simulink model "test_SOC_SOH"  (R2024a)
settings: Solver=VariableStepAuto  StartTime=0.0  StopTime=3600*24*7  RelTol=1e-3
values from neighbouring files (symbols this model uses):
  cell_capacity_nominal = 116.0    [CellDictionary.sldd]    (also in Gotion116CellDictionary.sldd)
  cycling_N_cycles : value not decoded    [TestDictionary.sldd]
  cycling_Q_change : value not decoded    [TestDictionary.sldd]
  lower_SOC = 0.0    [TestDictionary.sldd]
  R0_charge = 0.0011762548470330098 0.00082374580425955042 0.000528220046847626 0.00036375900896813311 0.0010441063780583621 0.00072163805067231468 0.00050986311152455624 0.00035574030260694049 0.0010321299216333078 0.00071105826266249655 0.00048266835826310457 0.00035372216488075841 0.001024720077996646 0.00069001121087368356 0.00048481817133183287 0.00034648647498852108 0.001011799939308299 0.0006697964359567    [CellDictionary.sldd]    (also in Gotion116CellDictionary.sldd)
  R0_discharge = 0.0011713156680267826 0.00080379131757867114 0.00053584971835591568 0.00037332457313021659 0.0011487629449379545 0.00077055056377129218 0.00052328698011887883 0.00035835507369999319 0.0011266444560462821 0.0007386844798434178 0.00050172364877783509 0.0003498356430994423 0.0010850138368129973 0.00069989297656780321 0.00047637432800705728 0.00034196489943770015 0.0010386918064711587 0.00065988337212    [CellDictionary.sldd]    (also in Gotion116CellDictionary.sldd)
  R1_charge = 0.00046991497657839924 0.0010779816764740048 0.00013720748025427109 0.00054498496863974164 0.00046376138253324481 0.00066376489201272156 0.00013720748025427109 0.00018528267520728436 0.00041621818829090906 0.00049349026745049 0.00020770204245624234 0.00018502550552971592 0.00041621893904479396 0.00049355079737852447 0.00036345316071937457 0.00018502550475278616 0.00030655167459223354 0.00020155261    [CellDictionary.sldd]    (also in Gotion116CellDictionary.sldd)
  R1_discharge = 0.00062343910396692745 0.00088344565476029683 0.000473998175802181 0.00030361323697364274 0.00034635505775940415 0.00063103261054306924 0.0003646139813862931 0.00025301103081136895 0.00024739646982814583 0.00052586050878589109 0.00030384498448857757 0.00023001002801033537 0.00022490588166195074 0.00047805500798717366 0.00027622271317143414 0.00021905716953365273 0.00022546269140634405 0.0003001510    [CellDictionary.sldd]    (also in Gotion116CellDictionary.sldd)
  R2_charge = 0.0013071970907491625 0.0011565350014947392 0.00094770363400168442 0.00027803074491849166 0.0011296066387324344 0.00079964133367552734 0.000585621349864987 0.00040094855176715479 0.00096825717163721565 0.00071275071905804873 0.00050086266287882315 0.00022186351951754667 0.000858047601085684 0.00068372107937354906 0.00048716119953890212 0.00021951334854306714 0.00082371775210131749 0.00056587719522    [CellDictionary.sldd]    (also in Gotion116CellDictionary.sldd)
  R2_discharge = 0.0082023616629522487 0.00477357645651923 0.0013535754139770782 0.00071689319983068869 0.0027341205543174162 0.0015911921521730766 0.00084598463373567378 0.00044805824989418042 0.0013670602771587081 0.00088399564009615365 0.00060427473838262416 0.00037338187491181703 0.00091137351810580548 0.00073666303341346137 0.00050356228198552015 0.0003556017856303019 0.00092980892733805819 0.0007515620058816    [CellDictionary.sldd]    (also in Gotion116CellDictionary.sldd)
  R3_charge = 0.0022791079484232404 0.00076358338365525792 0.0012549156736722906 0.00058631541275341111 0.0012276125164720909 0.00076358338365525792 0.00035824943217463234 0.00076079543468179163 0.0011171764499634 0.00069457337864931717 0.00035533139001579984 0.00094337886181821427 0.0006671085355807189 0.00046891528577433023 0.00033689307388307945 0.00072524071500878735 0.00058184070468519759 0.000371910545995    [CellDictionary.sldd]    (also in Gotion116CellDictionary.sldd)
  R3_discharge = 0.5961801788597515 0.049373498218042031 0.0017231068556688191 0.0031135501588106253 0.05961801788597515 0.0098746996436084068 0.00086155342783440954 0.0017297500882281251 0.0059618017885975146 0.0019749399287216814 0.00057436895188960632 0.0012355357773058038 0.000993633631432919 0.00065831330957389386 0.0004418222706843125 0.0011232143430052761 0.0013277019879200426 0.00096507261335108377 0.00043    [CellDictionary.sldd]    (also in Gotion116CellDictionary.sldd)
  soc_init = 0.31    [SOC_tester.m]    (also in TestDictionary.sldd = 0.5
                real
                1.0 1.0
           )
  Ts = 1.0    [EstimatorsDictionary.sldd]    (also in batteryStateTransition.m = u(3))
  upper_SOC = 1.0    [TestDictionary.sldd]
undefined symbols (not defined in the file or in its folder): R, thermal_mass
libraries: fl_lib x8, nesl_utility x4, simulink x3, BatteryEstimators x2, batteryecm_lib x1, batt_lib x1
settings Model: DataDictionary=TestDictionary.sldd  Creator=mmackenzie  LastModifiedBy=mmackenzie

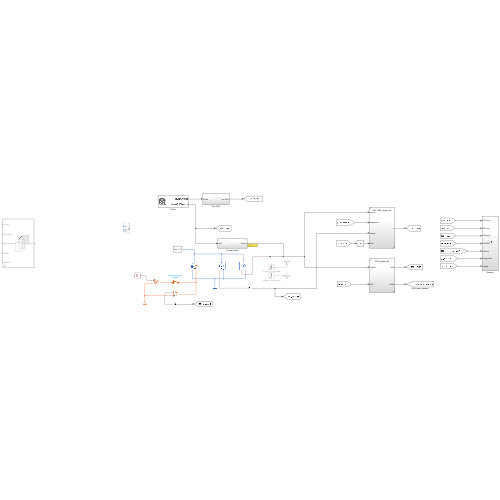
[thumbnail: Simulink's stored preview of the top-level diagram]
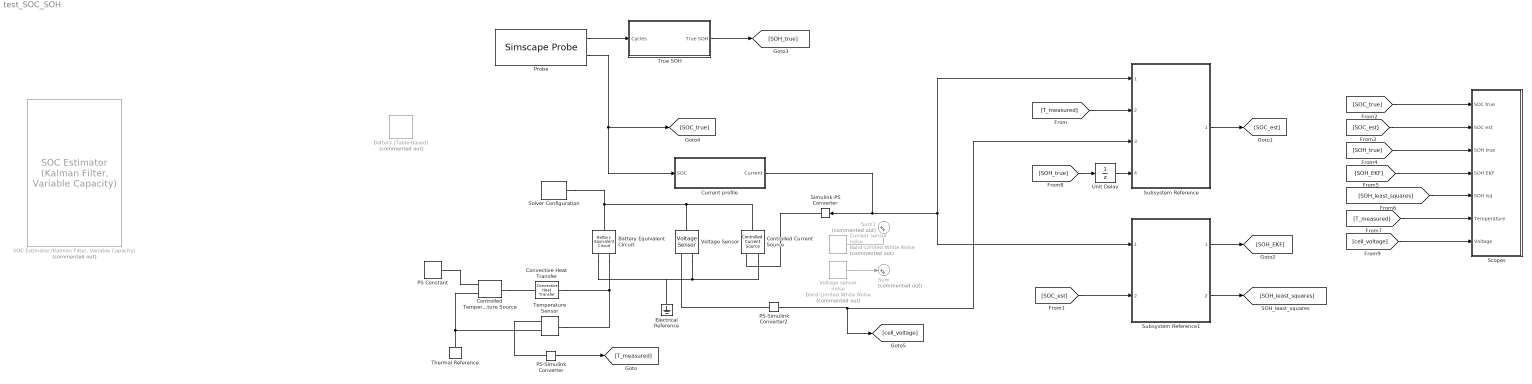
== system test_SOC_SOH ==
  Battery (Table-Based) : batteryecm_lib/Battery (Table-Based)  Commented=on  SOC_vec=SOC_vec  T_dependence=simscape.enum.tablebattery.temperature_dependence.yes  prm_dir=simscape.enum.tablebattery.prm_dir.noCurrentDirectionality  T_vec=T_vec K  V0_mat=V0_mat V  V0_vec=[3.5057, 3.566, 3.6337, 3.7127, 3.9259, 4.0777, 4.1928] V  V_range=[0, inf] V  R0_mat=R0_mat Ohm  R0_vec=[.0085, .0085, .0087, .0082, .0083, .0085, .0085] Ohm  R0_dis_mat=[.0117, .0085, .009; .011, .0085, .009; .0114, .0087, .0092; .0107, .0082, .0088; .0107, .0083, .0091; .0113, .0085, .0089; .0116, .0085, .0089] Ohm  R0_dis_vec=[.0085, .0085, .0087, .0082, .0083, .0085, .0085] Ohm  R0_ch_mat=[.0117, .0085, .009; .011, .0085, .009; .0114, .0087, .0092; .0107, .0082, .0088; .0107, .0083, .0091; .0113, .0085, .0089; .0116, .0085, .0089] Ohm  R0_ch_vec=[.0085, .0085, .0087, .0082, .0083, .0085, .0085] Ohm  AH=cell_capacity_init A*hr  prm_leak=simscape.enum.tablebattery.prm_leak.disabled  Rleak_vec=[8000, 7000, 6000] Ohm  Rleak=7e3 Ohm  extrapolation_option=simscape.enum.extrapolation.linear  SOC_port=simscape.enum.tablebattery.enable.yes  prm_dyn=simscape.enum.tablebattery.prm_dyn.rc1  R1_mat=R1_mat Ohm  R1_vec=[.0029, .0024, .0026, .0016, .0023, .0018, .0017] Ohm  tau1_mat=tau1_mat s  tau1_vec=[36, 45, 105, 29, 77, 33, 39] s  R2_mat=[.0109, .0029, .0013; .0069, .0024, .0012; .0047, .0026, .0013; .0034, .0016, .001; .0033, .0023, .0014; .0033, .0018, .0011; .0028, .0017, .0011] Ohm  R2_vec=[.0029, .0024, .0026, .0016, .0023, .0018, .0017] Ohm  tau2_mat=[20, 36, 39; 31, 45, 39; 109, 105, 61; 36, 29, 26; 59, 77, 67; 40, 33, 29; 25, 39, 33] s  tau2_vec=[36, 45, 105, 29, 77, 33, 39] s  R3_mat=[.0109, .0029, .0013; .0069, .0024, .0012; .0047, .0026, .0013; .0034, .0016, .001; .0033, .0023, .0014; .0033, .0018, .0011; .0028, .0017, .0011] Ohm  R3_vec=[.0029, .0024, .0026, .0016, .0023, .0018, .0017] Ohm  tau3_mat=[20, 36, 39; 31, 45, 39; 109, 105, 61; 36, 29, 26; 59, 77, 67; 40, 33, 29; 25, 39, 33] s  tau3_vec=[36, 45, 105, 29, 77, 33, 39] s  R4_mat=[.0109, .0029, .0013; .0069, .0024, .0012; .0047, .0026, .0013; .0034, .0016, .001; .0033, .0023, .0014; .0033, .0018, .0011; .0028, .0017, .0011] Ohm  R4_vec=[.0029, .0024, .0026, .0016, .0023, .0018, .0017] Ohm  tau4_mat=[20, 36, 39; 31, 45, 39; 109, 105, 61; 36, 29, 26; 59, 77, 67; 40, 33, 29; 25, 39, 33] s  tau4_vec=[36, 45, 105, 29, 77, 33, 39] s  R5_mat=[.0109, .0029, .0013; .0069, .0024, .0012; .0047, .0026, .0013; .0034, .0016, .001; .0033, .0023, .0014; .0033, .0018, .0011; .0028, .0017, .0011] Ohm  R5_vec=[.0029, .0024, .0026, .0016, .0023, .0018, .0017] Ohm  tau5_mat=[20, 36, 39; 31, 45, 39; 109, 105, 61; 36, 29, 26; 59, 77, 67; 40, 33, 29; 25, 39, 33] s  tau5_vec=[36, 45, 105, 29, 77, 33, 39] s  prm_fade=simscape.enum.tablebattery.prm_fade.tableN  N0=100  dV0=0  dR0=0  dAH=0  dRleak=0  dR1=0  dR2=0  dR3=0  dR4=0  dR5=0  N0vec=N0vec  Tfadevec=[298.15, 323.15] K  dV0vec=[0, 0, 0, 0, 0]  dR0vec=[0, 0, 0, 0, 0]  dAHvec=dAHvec  dRleakvec=[0, 0, 0, 0]  dR1vec=[0, 0, 0, 0, 0]  dR2vec=[0, 0, 0, 0]  dR3vec=[0, 0, 0, 0]  dR4vec=[0, 0, 0, 0]  dR5vec=[0, 0, 0, 0]  dV0mat=[0, 0; 0, 0; 0, 0; 0, 0]  dR0mat=[0, 0; 0, 0; 0, 0; 0, 0]  dAHmat=[0, 0; 0, 0; 0, 0; 0, 0]  dRleakmat=[0, 0; 0, 0; 0, 0; 0, 0]  dR1mat=[0, 0; 0, 0; 0, 0; 0, 0]  dR2mat=[0, 0; 0, 0; 0, 0; 0, 0]  dR3mat=[0, 0; 0, 0; 0, 0; 0, 0]  dR4mat=[0, 0; 0, 0; 0, 0; 0, 0]  dR5mat=[0, 0; 0, 0; 0, 0; 0, 0]  prm_age_modeling=simscape.enum.tablebattery.prm_age_modeling.equation  storage_dt_age_vec=[0] d  storage_T_age_vec=[273] K  prm_age_OCV=simscape.enum.tablebattery.prm_age_OCV.OCV  OCV_age=0.9  SOC_age=0.6  prm_age_resistance=simscape.enum.tablebattery.prm_age.disabled  OCV_scaling_age_resistance=2.2134e6  OCV_offset_age_resistance=1.632e6  temp_exp_age_resistance=0.515833569 V  t_exp_age_resistance=0.75  T_age_vec_resistance=[273.15, 298.15, 323.15] K  dt_age_vec_resistance=[0, 90, 180, 270] d  dR0_age_vec=[0, 0, 0]  t_meas_dR0_age=100 d  dR0_age_mat=[0, 0, 0; 0, 0, 0; 0, 0, 0; 0, 0, 0]  prm_age_capacity=simscape.enum.tablebattery.prm_age.disabled  OCV_scaling_age_capacity=1.5097e07  OCV_offset_age_capacity=8.3625e06  temp_exp_age_capacity=0.6011 V  t_exp_age_capacity=0.75  T_age_vec_capacity=[273.15, 298.15, 323.15] K  dt_age_vec_capacity=[0, 90, 180, 270] d  dAH_age_vec=[0, 0, 0]  t_meas_dAH_age=100 d  dAH_age_mat=[0, 0, 0; 0, 0, 0; 0, 0, 0; 0, 0, 0]  thermal_port=simscape.enum.thermaleffects.model  temperature=298.15 K  thermal_mass=thermal_mass*1.5 J/K  i_specify=off  i_priority=None  i=0 A  i_nominal_specify=off  i_nominal_value=1  i_nominal_unit=A  v_specify=off  v_priority=None  v=0 V  v_nominal_specify=off  v_nominal_value=1  v_nominal_unit=V  stateOfCharge_specify=on  stateOfCharge_priority=High  stateOfCharge=initialSOC  stateOfCharge_nominal_specify=off  stateOfCharge_nominal_value=1  stateOfCharge_nominal_unit=1  num_cycles_specify=off  num_cycles_priority=High  num_cycles=0  num_cycles_nominal_specify=off  num_cycles_nominal_value=1  num_cycles_nominal_unit=1  cell_temperature_specify=off  cell_temperature_priority=High  cell_temperature=298.15 K  cell_temperature_nominal_specify=off  cell_temperature_nominal_value=1  cell_temperature_nominal_unit=K
      settings: LibrarySourceBlock=|
      | batt_lib/Cells/Battery
      | (Table-Based)
  Battery Equivalent Circuit : batt_lib/Cells/Battery Equivalent Circuit  BatteryCapacity=cell_capacity_nominal A*hr  ThermalModel=simscape.battery.enum.cells.BatteryThermalModel.LumpedThermalMass  ExtrapolationMethod=simscape.enum.extrapolation.nearest  EnableFaultExotherm=false  TriggerTemperature=350 K  SOCBreakpoints=OCV_SOC  TemperatureBreakpoints=OCV_T degC  OpenCircuitVoltage=[3.5057, 3.566, 3.6337, 3.7127, 3.9259, 4.0777, 4.1928] V  OpenCircuitVoltageThermal=OCV_V V  VoltageRange=[2.8, 4.25] V  HysteresisModel=simscape.battery.enum.cells.HysteresisModel.none  MaximumHysteresisVoltage=[0, 0, 0, 0, 0, 0, 0] V  InstantaneousHysteresisVoltage=[0, 0, 0, 0, 0, 0, 0] V  HysteresisRate=0.1  MaximumHysteresisVoltageThermal=[0, 0, 0; 0, 0, 0; 0, 0, 0; 0, 0, 0; 0, 0, 0; 0, 0, 0; 0, 0, 0] V  InstantaneousHysteresisVoltageThermal=[0, 0, 0; 0, 0, 0; 0, 0, 0; 0, 0, 0; 0, 0, 0; 0, 0, 0; 0, 0, 0] V  HysteresisRateThermal=0.1  ResistanceSOCBreakpoints=ECM_SOC'  ResistanceTemperatureBreakpoints=ECM_T' degC  CurrentDirectionality=simscape.battery.enum.cells.BatteryEnable.Enabled  R0=[.0085, .0085, .0087, .0082, .0083, .0085, .0085] Ohm  R0Thermal=[.0117, .0085, .009; .011, .0085, .009; .0114, .0087, .0092; .0107, .0082, .0088; .0107, .0083, .0091; .0113, .0085, .0089; .0116, .0085, .0089] Ohm  DischargeR0=[.0085, .0085, .0087, .0082, .0083, .0085, .0085] Ohm  ChargeR0=[.0085, .0085, .0087, .0082, .0083, .0085, .0085] Ohm  ChargeR0Thermal=R0_charge' Ohm  DischargeR0Thermal=R0_discharge' Ohm  SelfDischargeResistor=simscape.battery.enum.cells.BatteryEnable.Disabled  SelfDischargeR=7e3 Ohm  SelfDischargeRThermal=[8000, 7000, 6000] Ohm  RCPairs=simscape.battery.enum.cells.RCPairs.rc3  R1=[.0029, .0024, .0026, .0016, .0023, .0018, .0017] Ohm  Tau1=[36, 45, 105, 29, 77, 33, 39] s  R2=[.0029, .0024, .0026, .0016, .0023, .0018, .0017] Ohm  Tau2=[36, 45, 105, 29, 77, 33, 39] s  R3=[.0029, .0024, .0026, .0016, .0023, .0018, .0017] Ohm  Tau3=[36, 45, 105, 29, 77, 33, 39] s  DischargeR1=[.0029, .0024, .0026, .0016, .0023, .0018, .0017] Ohm  DischargeTau1=[36, 45, 105, 29, 77, 33, 39] s  ChargeR1=[.0029, .0024, .0026, .0016, .0023, .0018, .0017] Ohm  ChargeTau1=[36, 45, 105, 29, 77, 33, 39] s  DischargeR2=[.0029, .0024, .0026, .0016, .0023, .0018, .0017] Ohm  DischargeTau2=[36, 45, 105, 29, 77, 33, 39] s  ChargeR2=[.0029, .0024, .0026, .0016, .0023, .0018, .0017] Ohm  ChargeTau2=[36, 45, 105, 29, 77, 33, 39] s  DischargeR3=[.0029, .0024, .0026, .0016, .0023, .0018, .0017] Ohm  DischargeTau3=[36, 45, 105, 29, 77, 33, 39] s  ChargeR3=[.0029, .0024, .0026, .0016, .0023, .0018, .0017] Ohm  ChargeTau3=[36, 45, 105, 29, 77, 33, 39] s  R1Thermal=[.0109, .0029, .0013; .0069, .0024, .0012; .0047, .0026, .0013; .0034, .0016, .001; .0033, .0023, .0014; .0033, .0018, .0011; .0028, .0017, .0011] Ohm  Tau1Thermal=[20, 36, 39; 31, 45, 39; 109, 105, 61; 36, 29, 26; 59, 77, 67; 40, 33, 29; 25, 39, 33] s  R2Thermal=[.0109, .0029, .0013; .0069, .0024, .0012; .0047, .0026, .0013; .0034, .0016, .001; .0033, .0023, .0014; .0033, .0018, .0011; .0028, .0017, .0011] Ohm  Tau2Thermal=[20, 36, 39; 31, 45, 39; 109, 105, 61; 36, 29, 26; 59, 77, 67; 40, 33, 29; 25, 39, 33] s  R3Thermal=[.0109, .0029, .0013; .0069, .0024, .0012; .0047, .0026, .0013; .0034, .0016, .001; .0033, .0023, .0014; .0033, .0018, .0011; .0028, .0017, .0011] Ohm  Tau3Thermal=[20, 36, 39; 31, 45, 39; 109, 105, 61; 36, 29, 26; 59, 77, 67; 40, 33, 29; 25, 39, 33] s  DischargeR1Thermal=R1_discharge' Ohm  DischargeTau1Thermal=R1_discharge' .* C1_discharge' s  ChargeR1Thermal=R1_charge' Ohm  ChargeTau1Thermal=R1_charge' .* C1_charge' s  DischargeR2Thermal=R2_discharge' Ohm  DischargeTau2Thermal=R2_discharge' .* C2_discharge' s  ChargeR2Thermal=R2_charge' Ohm  ChargeTau2Thermal=R2_charge' .* C2_charge' s  DischargeR3Thermal=R3_discharge' Ohm  DischargeTau3Thermal=R3_discharge' .* C3_discharge' s  ChargeR3Thermal=R3_charge' Ohm  ChargeTau3Thermal=R3_charge' .* C3_charge' s  CyclingAgingMethod=simscape.battery.enum.cells.CyclingAgingMethod.tableN  NumDisCycles=100  OCVChange=0  R0Change=0  CapacityChange=0  SelfDischargeRChange=0  R1Change=0  R2Change=0  R3Change=0  NumDisCyclesBreakpoints=cycling_N_cycles  AgingTemperatureBreakpoints=[298.15, 323.15] K  OCVChangeVec=cycling_OCV_change  R0ChangeVec=cycling_R0_change  CapacityChangeVec=cycling_Q_change  SelfDischargeRChangeVec=[0, 0, 0, 0]  R1ChangeVec=cycling_R1_change  R2ChangeVec=cycling_R2_change  R3ChangeVec=cycling_R3_change  OCVChangeThermal=[0, 0; 0, 0; 0, 0; 0, 0]  R0ChangeThermal=[0, 0; 0, 0; 0, 0; 0, 0]  CapacityChangeThermal=[0, 0; 0, 0; 0, 0; 0, 0]  SelfDischargeRChangeThermal=[0, 0; 0, 0; 0, 0; 0, 0]  R1ChangeThermal=[0, 0; 0, 0; 0, 0; 0, 0]  R2ChangeThermal=[0, 0; 0, 0; 0, 0; 0, 0]  R3ChangeThermal=[0, 0; 0, 0; 0, 0; 0, 0]  CalendarAgeResistance=simscape.battery.enum.cells.BatteryEnable.Disabled  CalendarAgeCapacity=simscape.battery.enum.cells.BatteryEnable.Disabled  CalendarAgingMethod=simscape.battery.enum.cells.CalendarAgingMethod.equation  StorageVariable=simscape.battery.enum.cells.StorageVariable.OCV  OCVDuringStorage=0.9  SOCDuringStorage=0.6  StorageTimeIntervals=[0] d  StorageTemperatures=[273] K  ResistanceScalingOCV=2.2134e6  ResistanceScalingOCVOffset=1.632e6  ResistanceExponentialIncrease=0.515833569 V  ResistanceTimeExponent=0.75  ResistanceAgeTemperatureBreakpoints=[273.15, 298.15, 323.15] K  ResistanceAgeTimeBreakpoints=[0, 90, 180, 270] d  PercentResistanceChange=[0, 0, 0]  ResistanceTimeBreakpoints=100 d  PercentResistanceChangeThermal=[0, 0, 0; 0, 0, 0; 0, 0, 0; 0, 0, 0]  CapacityScalingOCV=1.5097e07  CapacityScalingOCVOffset=8.3625e06  CapacityExponentialIncrease=0.6011 V  CapacityTimeExponent=0.75  CapacityAgeTemperatureBreakpoints=[273.15, 298.15, 323.15] K  CapacityAgeTimeBreakpoints=[0, 90, 180, 270] d  PercentCapacityChange=[0, 0, 0]  CapacityTimeBreakpoints=100 d  PercentCapacityChangeThermal=[0, 0, 0; 0, 0, 0; 0, 0, 0; 0, 0, 0]  SimulationTemperature=298.15 K  BatteryThermalMass=cell_thermal_mass J/K  ReversibleHeatModel=simscape.battery.enum.cells.ReversibleHeatModel.Disabled  EntropicCoefficient=[0, 0, 0, 0, 0, 0, 0] mV/K  AddedResistance=1e5 Ohm  ShortedResistance=1e-6 Ohm  ExothermModel=simscape.battery.enum.cells.ExothermModel.analytical  TabulateWithSOC=false  SOCvecExotherm=[0, .5, 1]  CurrInterruptTempSOC=[420, 420, 420] K  TotalHeatOfReactionSOC=[23000, 23000, 23000] J  CurrentInterruptTemperature=420 K  TotalHeatOfReaction=23e3 J  ExothermOnsetTemperature=350 K  ExothermOnsetTempSOC=[350, 350, 350] K  OnsetTempRate=0.02 K/min  ActivationEnergy=160e3 J/mol  ActivationEnergySOC=[160000, 160000, 160000] J/mol  ReactionOrder=1  ReactionOrderSOC=[1, 1, 1]  TemperaturesFromARC=[323, 373, 423, 438, 463, 483, 513, 543, 545, 547, 549, 551, 553, 573, 623, 773, 923, 943, 1003, 1063, 1113, 1123, 1133, 1153, 1173] K  TemperatureRatesFromARC=[.0001, .001, .025, .2, .4, .6, 1.1, 1.3, 1.9, 3, 5, 11.6, 183.3, 191.6, 200, 208.3, 200, 175, 8.33, 1.33, .33, .2, .13, .0017, .00017] K/s  TempRateVecARCSOC=repmat([.0001, .001, .025, .2, .4, .6, 1.1, 1.3, 1.9, 3, 5, 11.6, 183.3, 191.6, 200, 208.3, 200, 175, 8.33, 1.33, .33, .2, .13, .0017, .00017]', 1, 3) K/s  PercentThermalMassVented=40  PercentThermalMassVentedSOC=[40, 40, 40]  EnableFaultAddRes=false  EnableFaultShort=false  faultTriggerType=simscape.fault.triggertype.external  stateOfCharge_specify=on  stateOfCharge_priority=High  stateOfCharge=soc_init  stateOfCharge_nominal_specify=off  stateOfCharge_nominal_value=1  stateOfCharge_nominal_unit=1  numCycles_specify=off  numCycles_priority=High  numCycles=0  numCycles_nominal_specify=off  numCycles_nominal_value=1  numCycles_nominal_unit=1  batteryVoltage_specify=off  batteryVoltage_priority=None  batteryVoltage=0 V  batteryVoltage_nominal_specify=off  batteryVoltage_nominal_value=1  batteryVoltage_nominal_unit=V  batteryCurrent_specify=off  batteryCurrent_priority=None  batteryCurrent=0 A  batteryCurrent_nominal_specify=off  batteryCurrent_nominal_value=1  batteryCurrent_nominal_unit=A  batteryTemperature_specify=off  batteryTemperature_priority=High  batteryTemperature=298.15 K  batteryTemperature_nominal_specify=off  batteryTemperature_nominal_value=1  batteryTemperature_nominal_unit=K  hysteresisState_specify=off  hysteresisState_priority=High  hysteresisState=0  hysteresisState_nominal_specify=off  hysteresisState_nominal_value=1  hysteresisState_nominal_unit=1  isExothermFaulted_specify=off  isExothermFaulted_priority=None  isExothermFaulted=0  isExothermFaulted_nominal_specify=off  isExothermFaulted_nominal_value=1  isExothermFaulted_nominal_unit=1  isCurrentInterruptionTempExceeded_specify=off  isCurrentInterruptionTempExceeded_priority=None  isCurrentInterruptionTempExceeded=0  isCurrentInterruptionTempExceeded_nominal_specify=off  isCurrentInterruptionTempExceeded_nominal_value=1  isCurrentInterruptionTempExceeded_nominal_unit=1  reactionHeatRate_specify=off  reactionHeatRate_priority=None  reactionHeatRate=0 W  reactionHeatRate_nominal_specify=off  reactionHeatRate_nominal_value=1  reactionHeatRate_nominal_unit=W  reactionExtent_specify=off  reactionExtent_priority=None  reactionExtent=0  reactionExtent_nominal_specify=off  reactionExtent_nominal_value=1  reactionExtent_nominal_unit=1
      settings: InternalSimscapePortConfiguration="{\"Bottom\":[],\"Left\":[{\"id\":\"p\",\"label\":\"+\",\"type\":\"foundation.electrical.electrical\"}],\"Right\":[{\"id\":\"n\",\"label\":\"-\",\"type\":\"foundation.electrical.electrical\"},{\"id\":\"H\",\"label\":\"H\",\"type\":\"foundation.thermal.thermal\"}],\"Top\":[]}"
  Controlled Temperature Source : fl_lib/Thermal/Thermal Sources/Controlled Temperature Source
  Controlled Current Source : fl_lib/Electrical/Electrical Sources/Controlled Current Source
  Convective Heat Transfer : fl_lib/Thermal/Thermal Elements/Convective Heat Transfer  thermal_type=foundation.enum.constant_variable.constant  area=cell_Atot m^2  heat_tr_coeff=h_conv W/(K*m^2)  min_heat_tr_coeff=1e-3 W/(K*m^2)  T_specify=off  T_priority=None  T=0 K  T_nominal_specify=off  T_nominal_value=1  T_nominal_unit=K  Q_specify=off  Q_priority=None  Q=0 W  Q_nominal_specify=off  Q_nominal_value=1  Q_nominal_unit=W
  Current profile : Subsystem
  Current sensor noise : simulink/Sources/Band-Limited White Noise  Commented=on  Cov=1e-3/5  Ts=1  seed=1234
  Electrical Reference : fl_lib/Electrical/Electrical Elements/Electrical Reference
  PS Constant : fl_lib/Physical Signals/Sources/PS Constant  constant=298.15
  PS-Simulink Converter : nesl_utility/PS-Simulink Converter  PhysicalDomain=network_engine_domain  SubClassName=ps_output  LeftPortType=input  RightPortType=output  PseudoPeriodic=off  Frequencies=[]  VectorFormat=inherit  Unit=inherit  AffineConversion=off
  PS-Simulink Converter2 : nesl_utility/PS-Simulink Converter  PhysicalDomain=network_engine_domain  SubClassName=ps_output  LeftPortType=input  RightPortType=output  PseudoPeriodic=off  Frequencies=[]  VectorFormat=inherit  Unit=inherit  AffineConversion=off
  Probe : SimscapeProbe  BoundBlock=14  Variables={numCycles, stateOfCharge}
  "SOC Estimator (Kalman Filter, Variable Capacity)" : BatteryEstimators/SOC Estimator (Kalman Filter, Variable Capacity)  Commented=on  CurrentInputPartition=off  filterType=Extended Kalman filter  alpha=1  beta=2  kappa=0  Q=Q  Q_2RC=|  R=R  P0=P0  P0_2RC=[1e-5 0 0; 0 1 0;0 0 1]  Ts=Ts  chargeDynamics=One time-constant dynamics  SOC_vec=SOC_vec  T_vec=T_vec  R0_mat=R0_mat  R1_mat=R1_mat  tau1_mat=tau1_mat  R2_mat=[.0109, .0029, .0013; .0069, .0024, .0012; .0047, .0026, .0013; .0034, .0016, .001; .0033, .0023, .0014; .0033, .0018, .0011; .0028, .0017, .0011]  tau2_mat=[20, 36, 39; 31, 45, 39; 109, 105, 61; 36, 29, 26; 59, 77, 67; 40, 33, 29; 25, 39, 33]  V0_mat=V0_mat
      | [1e-6 0 0;
      | 0 1e-6 0;0 0 1e-6]
      settings: LibrarySourceBlock=|
      | batt_sl_lib/Estimators/SOC Estimator
      | (Kalman Filter, Variable Capacity)
  Scopes : Subsystem
  Simulink-PS Converter : nesl_utility/Simulink-PS Converter  PhysicalDomain=network_engine_domain  SubClassName=ps_input  LeftPortType=input  RightPortType=output  PseudoPeriodic=off  Frequencies=[]  NoiseDistribution=none  NoiseParameters=[]  Unit=1  AffineConversion=off  FilteringAndDerivatives=provide  SimscapeFilterOrder=1  InputFilterTimeConstant=0.001  UdotUserProvided=0
  Solver Configuration : nesl_utility/Solver Configuration  PhysicalDomain=network_engine_domain  SubClassName=solver  LeftPortType=input  RightPortType=generic  Tones=[]  Harmonics=[]  SimulateNoise=off  Profile=off  UseLocalSampling=off  EnableSwitchedLinearOptims=on  FrequencyDomain=off  UseCCode=off  RelTol=0.001  AbsTol=0.001  MinStep=1e-09  ToWorkspace=off  RevertToSquareIcSolve=off  NumHomotopyIterations=100  PhasorMode=off  PhasorModeNumHarmonics=1  ConsistencySolver=NEWTON_XTOL_AFTER_FTOL  IndexReductionMethod=DerivativeReplacement  DoDC=off  ResidualTolerance=1e-09  ConsistencyTolSource=GLOBAL  ConsistencyAbsTol=0.001  ConsistencyRelTol=0.001  ConsistencyTolFactor=0.001  UseLocalSolver=on  LocalSolverChoice=NE_BACKWARD_EULER_ADVANCER  ResolveIndetEquations=on  FunctionEvalNumThread=1  LocalSolverSampleTime=1  DoFixedCost=on  MaxNonlinIter=3  MaxModeIter=2  ComputeImpulses=off  ImpulseIterations=2  LinearAlgebra=auto  LinearAlgebraNumThread=0  EquationFormulation=NE_TIME_EF  DelaysMemoryBudget=1024  AutomaticFiltering=on  FilteringTimeConstant=0.001  PartitionStorageMethod=AS_NEEDED  PartitionMemoryBudget=1024  PartitionMethod=ROBUST  MultibodyUseLocalSolver=off  MultibodyLocalSolverChoice=ODE1  MultibodyLocalSolverSampleTime=0.001
  Subsystem Reference : Subsystem  ReferencedSubsystem=SOC_EKF_single_cell
      settings: PermitHierarchicalResolution=None
  Subsystem Reference1 : Subsystem  ReferencedSubsystem=SOH_single_cell
      settings: PermitHierarchicalResolution=None
  Sum : Sum  Commented=on  Inputs=|++
  Sum1 : Sum  Commented=on  Inputs=|++
  Temperature Sensor : fl_lib/Thermal/Thermal Sensors/Temperature Sensor  temperature_measure=foundation.enum.MeasurementReference.difference
  Thermal Reference : fl_lib/Thermal/Thermal Elements/Thermal Reference
  True SOH : Subsystem
  Unit Delay : UnitDelay  InitialCondition=1  SampleTime=-1  HasFrameUpgradeWarning=on
  Voltage Sensor : fl_lib/Electrical/Electrical Sensors/Voltage Sensor
  Voltage sensor noise : simulink/Sources/Band-Limited White Noise  Commented=on  Cov=1e-3/2  Ts=1  seed=1234
  wires:
  PS-Simulink Converter/1 -> [T_measured]
  Probe/2 -> Current profile/1(SOC), [SOC_true]
  Current profile/1(Current) -> Subsystem Reference/1, Subsystem Reference1/1, Simulink-PS Converter/1
  [T_measured] -> Subsystem Reference/2
  Subsystem Reference/1 -> [SOC_est]
  [SOC_est] -> Subsystem Reference1/2
  Subsystem Reference1/1 -> [SOH_EKF]
  Subsystem Reference1/2 -> [SOH_least_squares]
  True SOH/1(True SOH) -> [SOH_true]
  [SOC_true] -> Scopes/1(SOC true)
  [SOC_est] -> Scopes/2(SOC est)
  [SOH_true] -> Scopes/3(SOH true)
  [SOH_EKF] -> Scopes/4(SOH EKF)
  [SOH_least_squares] -> Scopes/5(SOH lsq)
  [T_measured] -> Scopes/6(Temperature)
  PS-Simulink Converter2/1 -> Subsystem Reference/3, [cell_voltage]
  Probe/1 -> True SOH/1(Cycles)
  [cell_voltage] -> Scopes/7(Voltage)
  Voltage sensor noise/1 -> Sum/1
  Current sensor noise/1 -> Sum1/2
  [SOH_true] -> Unit Delay/1
  Unit Delay/1 -> Subsystem Reference/4
  connections:
  Convective Heat Transfer/LConn1 -- Battery Equivalent Circuit/RConn2 -- Temperature Sensor/LConn1
  Controlled Temperature Source/LConn1 -- Convective Heat Transfer/RConn1
  Thermal Reference/LConn1 -- Controlled Temperature Source/RConn2 -- Temperature Sensor/RConn1
  PS-Simulink Converter/LConn1 -- Temperature Sensor/RConn2
  Voltage Sensor/LConn1 -- Solver Configuration/RConn1 -- Battery Equivalent Circuit/LConn1 -- Controlled Current Source/LConn1
  Voltage Sensor/RConn2 -- Controlled Current Source/RConn2 -- Battery Equivalent Circuit/RConn1 -- Electrical Reference/LConn1
  PS-Simulink Converter2/LConn1 -- Voltage Sensor/RConn1
  Simulink-PS Converter/RConn1 -- Controlled Current Source/RConn1
  PS Constant/RConn1 -- Controlled Temperature Source/RConn1

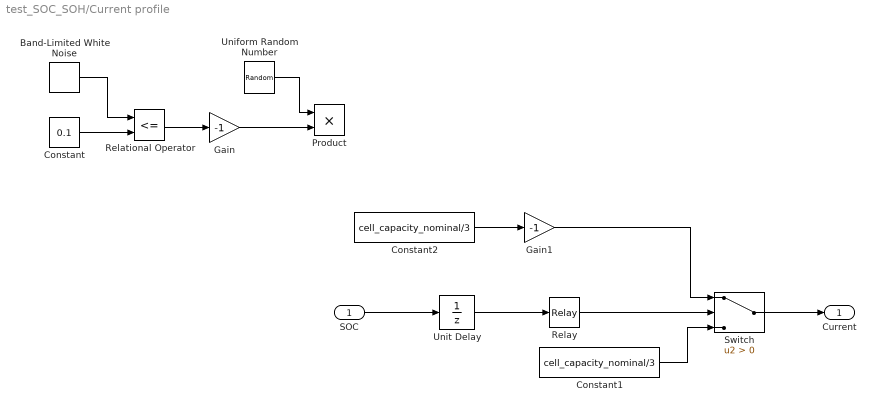
== system test_SOC_SOH/Current profile ==
  SOC : Inport
  Band-Limited White Noise : simulink/Sources/Band-Limited White Noise  Cov=[0.1]  Ts=0.1  seed=[23341]
  Constant : Constant  Value=0.1
  Constant1 : Constant  Value=cell_capacity_nominal/3
  Constant2 : Constant  Value=cell_capacity_nominal/3
  Gain : Gain  Gain=-1
  Gain1 : Gain  Gain=-1
  Product : Product
  Relational Operator : RelationalOperator  Operator=<=  OutDataTypeStr=boolean  RndMeth=Simplest  InputSameDT=off
  Relay : Relay  OnSwitchValue=upper_SOC  OffSwitchValue=lower_SOC  OffOutputValue=-1
  Switch : Switch  Criteria=u2 > Threshold  SaturateOnIntegerOverflow=off  InputSameDT=off
  Uniform Random Number : UniformRandomNumber  Minimum=5  Maximum=55  SampleTime=100
  Unit Delay : UnitDelay  InitialCondition=soc_init  SampleTime=-1  HasFrameUpgradeWarning=on
  Current : Outport
  wires:
  Switch/1 -> Current/1
  Constant/1 -> Relational Operator/2
  Relational Operator/1 -> Gain/1
  Uniform Random Number/1 -> Product/1
  Constant1/1 -> Switch/3
  Band-Limited White Noise/1 -> Relational Operator/1
  Unit Delay/1 -> Relay/1
  Relay/1 -> Switch/2
  Gain/1 -> Product/2
  SOC/1 -> Unit Delay/1
  Gain1/1 -> Switch/1
  Constant2/1 -> Gain1/1

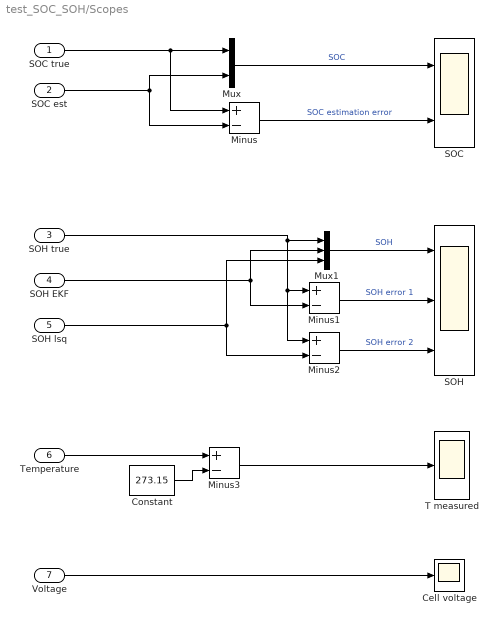
== system test_SOC_SOH/Scopes ==
  SOC true : Inport
  SOC est : Inport  Port=2
  SOH true : Inport  Port=3
  SOH EKF : Inport  Port=4
  SOH lsq : Inport  Port=5
  Temperature : Inport  Port=6
  Voltage : Inport  Port=7
  Cell voltage : Scope
  Constant : Constant  Value=273.15
  Minus{,1..3} (4 alike) : Sum  Inputs=+-
  Mux : Mux  Inputs=2
  Mux1 : Mux  Inputs=3
  SOC : Scope  NumInputPorts=2
  SOH : Scope  NumInputPorts=3
  T measured : Scope
  wires:
  Minus2/1 -> SOH/3  "SOH error 2"
  SOC est/1 -> Minus/2, Mux/2
  SOH true/1 -> Minus2/1, Minus1/1, Mux1/1
  SOC true/1 -> Minus/1, Mux/1
  SOH EKF/1 -> Mux1/2, Minus1/2
  SOH lsq/1 -> Mux1/3, Minus2/2
  Minus/1 -> SOC/2  "SOC estimation error"
  Minus1/1 -> SOH/2  "SOH error 1"
  Mux/1 -> SOC/1  "SOC"
  Mux1/1 -> SOH/1  "SOH"
  Temperature/1 -> Minus3/1
  Minus3/1 -> T measured/1
  Constant/1 -> Minus3/2
  Voltage/1 -> Cell voltage/1

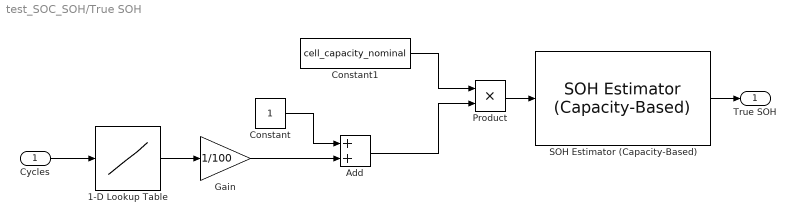
== system test_SOC_SOH/True SOH ==
  Cycles : Inport
  1-D Lookup Table : Lookup_n-D  NumberOfTableDimensions=1  BreakpointsForDimension1=cycling_N_cycles  Table=cycling_Q_change  InternalRulePriority=Speed  RndMeth=Simplest
  Add : Sum
  Constant : Constant
  Constant1 : Constant  Value=cell_capacity_nominal
  Gain : Gain  Gain=1/100
  Product : Product
  SOH Estimator (Capacity-Based) : BatteryEstimators/SOH Estimator (Capacity-Based)  AH_new=cell_capacity_nominal  AH_eol=1e-6
      settings: LibrarySourceBlock=batt_sl_lib/Estimators/SOH Estimator (Capacity-Based)
  True SOH : Outport
  wires:
  Product/1 -> SOH Estimator (Capacity-Based)/1
  Constant1/1 -> Product/1
  Add/1 -> Product/2
  Gain/1 -> Add/2
  Cycles/1 -> 1-D Lookup Table/1
  1-D Lookup Table/1 -> Gain/1
  Constant/1 -> Add/1
  SOH Estimator (Capacity-Based)/1 -> True SOH/1
